simulink model "model_CharakterystykaStatyczna"  (R2017a)
settings: Solver=ode45  StartTime=0.0  StopTime=200  MaxStep=1/60  RelTol=1e-6  EnableMultiTasking=on
undefined symbols (not defined in the file or in its folder): sigbuilder_block
libraries: simulink x1
settings Model: Creator=Krzys  LastModifiedBy=Szwank
settings DataIOCC: LimitDataPoints=on  SaveFormat=Array  SignalLoggingSaveFormat=ModelDataLogs
settings OptimizationCC: LifeSpan=inf
settings DebuggingCC: UnderspecifiedInitializationDetection=Classic  MergeDetectMultiDrivingBlocksExec=none  SolverPrmCheckMsg=warning  FcnCallInpInsideContextMsg=warning  StateNameClashWarn=warning  SFUnexpectedBacktrackingDiag=warning  SFNoUnconditionalDefaultTransitionDiag=warning  SFExecutionAtInitializationDiag=none
settings HardwareCC: ProdBitPerPointer=32  ProdBitPerSizeT=32  ProdBitPerPtrDiffT=32  ProdLargestAtomicFloat=None  ProdIntDivRoundTo=Undefined  ProdEndianess=Unspecified  ProdWordSize=32  ProdHWDeviceType=32-bit Generic
settings ModelReferenceCC: PropagateSignalLabelsOutOfModel=off
settings GRTTargetCC: TargetLangStandard=C89/C90 (ANSI)  CombineOutputUpdateFcns=off  GRTInterface=on
settings ConfigComp: CovMetricSettings=dw  CovHtmlReporting=on  CovSaveCumulativeToWorkspaceVar=on  CovSaveSingleToWorkspaceVar=on  CovExternalEMLEnable=off

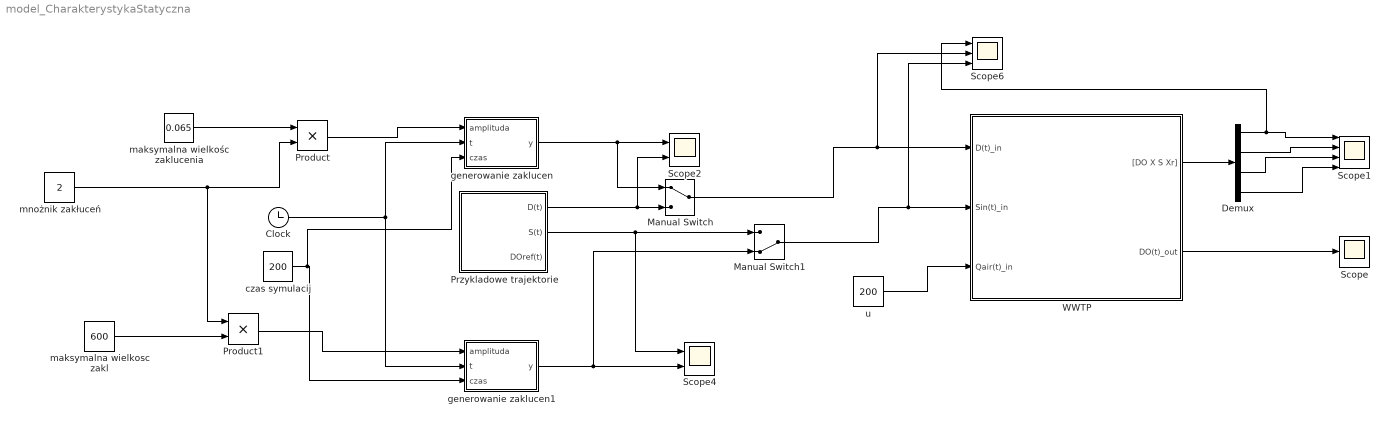
== system model_CharakterystykaStatyczna ==
  Clock : Clock
  Demux : Demux
  Manual Switch : ManualSwitch
  Manual Switch1 : ManualSwitch  CurrentSetting=0
  Product : Product
  Product1 : Product
  Przykladowe trajektorie : Subsystem  Tag=STV Subsys  LoadFcn=sigbuilder_block('load');  StartFcn=sigbuilder_block('start');  StopFcn=sigbuilder_block('stop');  ClipboardFcn=sigbuilder_block('clipboard');  mask(Sigbuilder block){tuvar=[0:10]}
      mask help: Sigbuilder GUI
      mask init:
      | if ~strcmp(get_param(bdroot(gcbh),'SimulationStatus'),'stopped') tuvar = sigbuilder_block('maskInit'); end
      settings: CopyFcn=sigbuilder_block('copy');  DeleteFcn=sigbuilder_block('delete');  ModelCloseFcn=sigbuilder_block('modelClose');  PreSaveFcn=sigbuilder_block('preSave');  PauseFcn=sigbuilder_block('pause')  ContinueFcn=sigbuilder_block('continue')  NameChangeFcn=sigbuilder_block('namechange');  OpenFcn=sigbuilder_block('open',[883.5 257.25 550.5 359.25 ]);  CloseFcn=sigbuilder_block('close');
      mask Display: plot(0, 0, 100, 100,[2, 2, 32, 32, 2], [68, 8, 8, 68, 68],[32, 2], [38, 38], [32, 19, 2],[53, 60, 44], [32, 17, 17, 2],[16, 16, 31, 31]);txt = getActiveGroup(gcbh);text(2, 100, txt,'verticalAlignment', 'top');
  Scope : Scope
  Scope1 : Scope  NumInputPorts=4
  Scope2 : Scope  NumInputPorts=2
  Scope4 : Scope  NumInputPorts=2
  Scope6 : Scope  NumInputPorts=3
  WWTP : Subsystem  mask{stateX=1225, stateS=20, stateDO=6, stateXr=2333}
  czas symulacij : Constant  Value=200
  generowanie zaklucen : MATLAB Function  TreatAsAtomicUnit=on
  "generowanie zaklucen1 " : MATLAB Function  TreatAsAtomicUnit=on
  "maksymalna wielkosc zakl " : Constant  Value=600
  "maksymalna wielkośc zaklucenia " : Constant  Value=0.065
  mnożnik zakłuceń : Constant  Value=2
  "u " : Constant  Value=200
  wires:
  WWTP/1("[DO X S Xr]") -> Demux/1
  Przykladowe trajektorie/1(D(t)) -> Scope2/2, Manual Switch/2
  Przykladowe trajektorie/2(S(t)) -> Manual Switch1/1, Scope4/1
  Manual Switch1/1 -> Scope6/3, WWTP/2(Sin(t)_in)
  Manual Switch/1 -> Scope6/2, WWTP/1(D(t)_in)
  "u "/1 -> WWTP/3(Qair(t)_in)
  WWTP/2(DO(t)_out) -> Scope/1
  Demux/1 -> Scope6/1, Scope1/1
  Demux/2 -> Scope1/2
  Demux/3 -> Scope1/3
  Demux/4 -> Scope1/4
  generowanie zaklucen/1(y) -> Manual Switch/1, Scope2/1
  Clock/1 -> "generowanie zaklucen1 "/2(t), generowanie zaklucen/2(t)
  "generowanie zaklucen1 "/1(y) -> Manual Switch1/2, Scope4/2
  "maksymalna wielkośc zaklucenia "/1 -> Product/1
  mnożnik zakłuceń/1 -> Product1/1, Product/2
  Product/1 -> generowanie zaklucen/1(amplituda)
  Product1/1 -> "generowanie zaklucen1 "/1(amplituda)
  "maksymalna wielkosc zakl "/1 -> Product1/2
  czas symulacij/1 -> generowanie zaklucen/3(czas), "generowanie zaklucen1 "/3(czas)

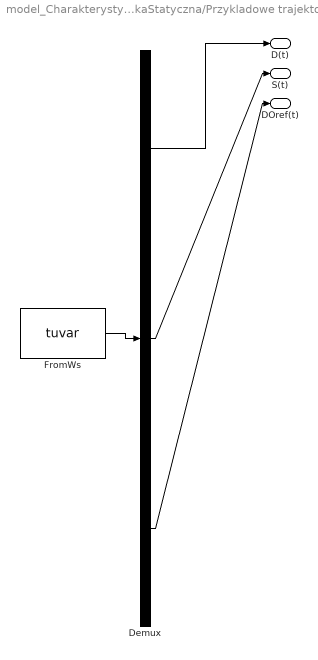
== system model_CharakterystykaStatyczna/Przykladowe trajektorie ==
  Demux : Demux  Tag=STV Demux  Outputs=3
  FromWs : FromWorkspace  Tag=STV FromWs  VariableName=tuvar  SampleTime=0
      SigBuilderData=|
      | common.afterFinalStr = 'Extrapolate'
      | common.sampleTime = 0
      | dataSet.timeRange = [0 24]
      | dataSet.name = 'Group 1'
      | sbobj.Groups.Name = 'Group 1'
      | sbobj.Groups.Signals(1).Name = 'D(t)'
      | sbobj.Groups.Signals(1).XData = [0 4 4 7 7 12 12 16 16 20 20 24]
      | sbobj.Groups.Signals(1).YData = [0.065 0.065 0.025 0.025 0.05 0.05 0.04 0.04 0.065 0.065 0.03 0.03]
      | sbobj.Groups.Signals(2).Name = 'S(t)'
      | sbobj.Groups.Signals(2).XData = [0 4 4 7 7 12 12 16 16 20 20 24]
      | sbobj.Groups.Signals(2).YData = [600 600 200 200 500 500 400 400 600 600 350 350]
      | sbobj.Groups.Signals(3).Name = 'DOref(t)'
      | sbobj.Groups.Signals(3).XData = [0 2 2 4 4 6 6 8 8 10 10 12 12 14 14 16 16 18 18 20 20 22 22 24]
      | sbobj.Groups.Signals(3).YData = [1.5 1.5 9.4 9.4 5 5 2 2 2.5 2.5 7 7 2.5 2.5 4 4 8.5 8.5 6 6 2 2 3 3]
      | sbobj.Groups.TimeRange = [0 24]
  D(t) : Outport  Tag=STV Outport
  S(t) : Outport  Tag=STV Outport  Port=2
  DOref(t) : Outport  Tag=STV Outport  Port=3
  wires:
  Demux/1 -> D(t)/1
  FromWs/1 -> Demux/1
  Demux/2 -> S(t)/1
  Demux/3 -> DOref(t)/1

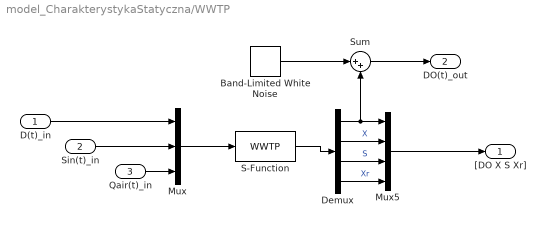
== system model_CharakterystykaStatyczna/WWTP ==
  D(t)_in : Inport
  Sin(t)_in : Inport  Port=2
  Qair(t)_in : Inport  Port=3
  Band-Limited White Noise : simulink/Sources/Band-Limited White Noise  Cov=[0.001]  Ts=1/60  seed=[23341]
  Demux : Demux
  Mux : Mux  Inputs=3
  Mux5 : Mux
  S-Function : S-Function  FunctionName=WWTP  Parameters=stateX stateS stateDO stateXr  SFunctionDeploymentMode=off  EnableBusSupport=off
  Sum : Sum  Inputs=|++
  "[DO X S Xr]" : Outport
  DO(t)_out : Outport  Port=2
  wires:
  D(t)_in/1 -> Mux/1
  Sin(t)_in/1 -> Mux/2
  Qair(t)_in/1 -> Mux/3
  Mux/1 -> S-Function/1
  S-Function/1 -> Demux/1
  Demux/2 -> Mux5/2  "X"
  Demux/3 -> Mux5/3  "S"
  Demux/4 -> Mux5/4  "Xr"
  Demux/1 -> Mux5/1, Sum/2
  Band-Limited White Noise/1 -> Sum/1
  Sum/1 -> DO(t)_out/1
  Mux5/1 -> "[DO X S Xr]"/1

== matlab function model_CharakterystykaStatyczna/generowanie zaklucen ==
  data: amplituda input; y output; t input; czas input
function y = fcn(amplituda,t,czas)

if(t<4/25*czas||(t >= 16/25*czas && t < 20/25*czas))
y = amplituda;
return
elseif(((t >= 4/25*czas && t < 7/25*czas)))
y = amplituda*0.025/0.065;
return
elseif(((t >= 7/25*czas && t < 12/25*czas)))
y = amplituda*0.05/0.065;
return
elseif(((t >= 12/25*czas && t < 16/25*czas)))
y = amplituda*0.04/0.065;
return
elseif(((t >= 20/25*czas && t < 25/25*czas)))
y = amplituda*0.03/0.065;
return
end
y=0;

== matlab function model_CharakterystykaStatyczna/generowanie zaklucen1  ==
  data: amplituda input; y output; t input; czas input
function y = fcn(amplituda,t,czas)

if(t<4/25*czas||(t >= 16/25*czas && t < 20/25*czas))
y = amplituda;
return

elseif(((t >= 4/25*czas && t < 7/25*czas)))
y = amplituda/3;
return

elseif(((t >= 7/25*czas && t < 12/25*czas)))
y = amplituda*0.83;
return

elseif(((t >= 12/25*czas && t < 16/25*czas)))
y = amplituda*2/3;
return

elseif(((t >= 20/25*czas && t < 25/25*czas)))
y = amplituda*0.58;
return

end
y=0;
